simulink subsystem "Reductor"  (R2023a)
settings: Solver=VariableStepAuto  StartTime=0.0  StopTime=10.0  RelTol=1e-3
model mask{i_gear=100, J_gear=2.4e-6, vis_friction_coef_gear=0.15}
values from neighbouring files (symbols this model uses):
  i_gear = 100    [const.m]
  J_gear = 2.4e-6    (= 2.4e-06)    [const.m]
  vis_friction_coef_gear = 0.003    [const.m]
settings Model: Creator=mrrom  LastModifiedBy=mrrom

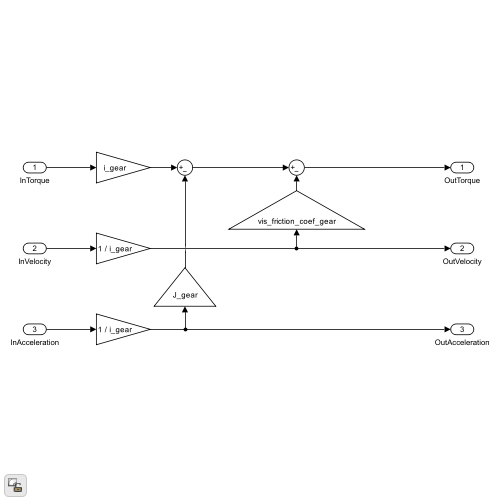
[thumbnail: Simulink's stored preview of the top-level diagram]
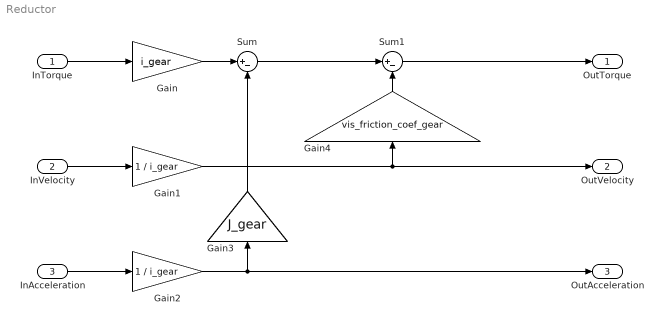
== system Reductor ==
  InTorque : Inport
  InVelocity : Inport  Port=2
  InAcceleration : Inport  Port=3
  Gain : Gain  Gain=i_gear
  Gain1 : Gain  Gain=1 / i_gear
  Gain2 : Gain  Gain=1 / i_gear
  Gain3 : Gain  Gain=J_gear
  Gain4 : Gain  Gain=vis_friction_coef_gear
  Sum : Sum  Inputs=|+-
  Sum1 : Sum  Inputs=|+-
  OutTorque : Outport
  OutVelocity : Outport  Port=2
  OutAcceleration : Outport  Port=3
  wires:
  Sum/1 -> Sum1/1
  Gain2/1 -> Gain3/1, OutAcceleration/1
  Gain1/1 -> Gain4/1, OutVelocity/1
  Gain4/1 -> Sum1/2
  InTorque/1 -> Gain/1
  Gain3/1 -> Sum/2
  InAcceleration/1 -> Gain2/1
  Sum1/1 -> OutTorque/1
  Gain/1 -> Sum/1
  InVelocity/1 -> Gain1/1
